simulink model "model"  (R2019b)
settings: Solver=VariableStepAuto  StartTime=0.0  StopTime=20.0  RelTol=1e-3
settings Model: Creator=szymo  LastModifiedBy=szymo

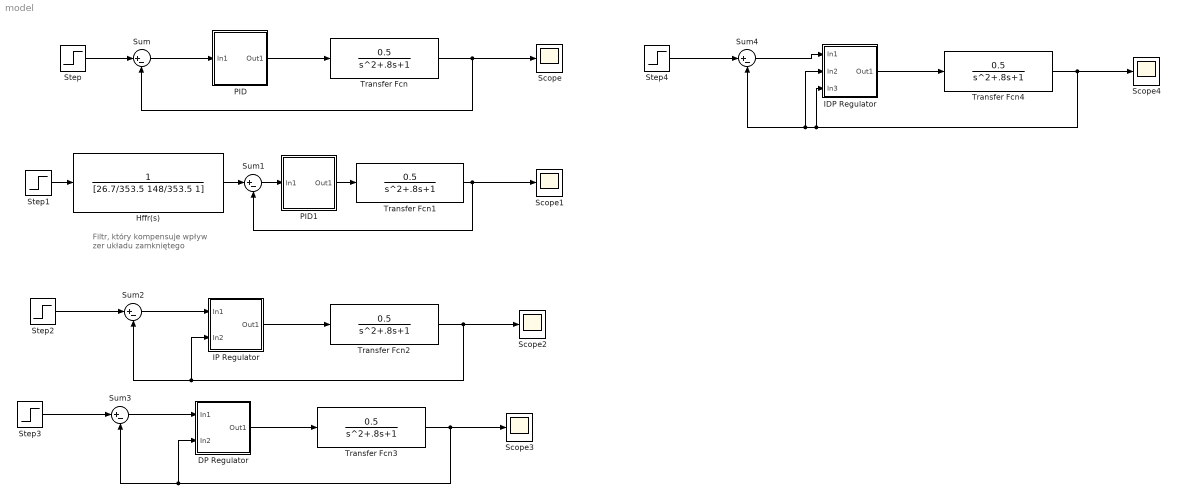
== system model ==
  note: Filtr, który kompensuje wpływ
      | zer układu zamkniętego
  DP Regulator : Subsystem
  Hffr(s) : TransferFcn  Denominator=[26.7/353.5 148/353.5 1]
  IDP Regulator : Subsystem
  IP Regulator : Subsystem
  PID : Subsystem
  PID1 : Subsystem
  Scope{,1..4} (5 alike) : Scope
  Step{,1..4} (5 alike) : Step  SampleTime=0
  Sum{,1..4} (5 alike) : Sum  Inputs=|+-
  Transfer Fcn{,1..4} (5 alike) : TransferFcn  Numerator=[0.5]  Denominator=[1 .8 1]
  wires:
  Transfer Fcn/1 -> Sum/2, Scope/1
  PID/1(Out1) -> Transfer Fcn/1
  Sum/1 -> PID/1(In1)
  Step/1 -> Sum/1
  Transfer Fcn1/1 -> Sum1/2, Scope1/1
  Sum1/1 -> PID1/1(In1)
  PID1/1(Out1) -> Transfer Fcn1/1
  Step1/1 -> Hffr(s)/1
  Hffr(s)/1 -> Sum1/1
  Step2/1 -> Sum2/1
  Sum2/1 -> IP Regulator/1(In1)
  IP Regulator/1(Out1) -> Transfer Fcn2/1
  Transfer Fcn2/1 -> IP Regulator/2(In2), Sum2/2, Scope2/1
  Step3/1 -> Sum3/1
  Transfer Fcn3/1 -> DP Regulator/2(In2), Sum3/2, Scope3/1
  Sum3/1 -> DP Regulator/1(In1)
  DP Regulator/1(Out1) -> Transfer Fcn3/1
  Sum4/1 -> IDP Regulator/1(In1)
  IDP Regulator/1(Out1) -> Transfer Fcn4/1
  Step4/1 -> Sum4/1
  Transfer Fcn4/1 -> IDP Regulator/3(In3), IDP Regulator/2(In2), Sum4/2, Scope4/1

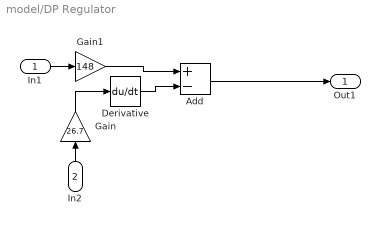
== system model/DP Regulator ==
  In1 : Inport
  In2 : Inport  Port=2
  Add : Sum  Inputs=+-
  Derivative : Derivative
  Gain : Gain  Gain=26.7
  Gain1 : Gain  Gain=148
  Out1 : Outport
  wires:
  In2/1 -> Gain/1
  Gain1/1 -> Add/1
  In1/1 -> Gain1/1
  Add/1 -> Out1/1
  Derivative/1 -> Add/2
  Gain/1 -> Derivative/1

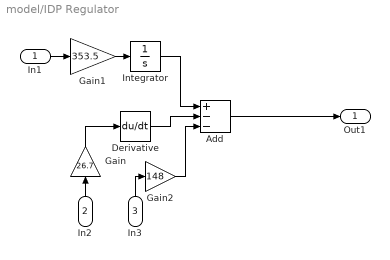
== system model/IDP Regulator ==
  In1 : Inport
  In2 : Inport  Port=2
  In3 : Inport  Port=3
  Add : Sum  Inputs=+--
  Derivative : Derivative
  Gain : Gain  Gain=26.7
  Gain1 : Gain  Gain=353.5
  Gain2 : Gain  Gain=148
  Integrator : Integrator
  Out1 : Outport
  wires:
  In2/1 -> Gain/1
  Add/1 -> Out1/1
  Derivative/1 -> Add/2
  Gain/1 -> Derivative/1
  In3/1 -> Gain2/1
  Gain2/1 -> Add/3
  In1/1 -> Gain1/1
  Gain1/1 -> Integrator/1
  Integrator/1 -> Add/1

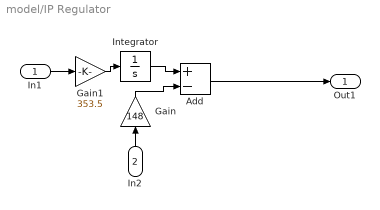
== system model/IP Regulator ==
  In1 : Inport
  In2 : Inport  Port=2
  Add : Sum  Inputs=+-
  Gain : Gain  Gain=148
  Gain1 : Gain  Gain=353.5
  Integrator : Integrator
  Out1 : Outport
  wires:
  In2/1 -> Gain/1
  Gain/1 -> Add/2
  Gain1/1 -> Integrator/1
  Integrator/1 -> Add/1
  In1/1 -> Gain1/1
  Add/1 -> Out1/1

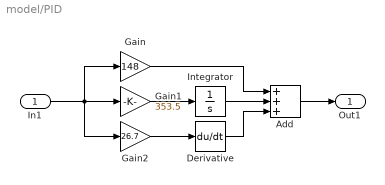
== system model/PID ==
  In1 : Inport
  Add : Sum  Inputs=+++
  Derivative : Derivative
  Gain : Gain  Gain=148
  Gain1 : Gain  Gain=353.5
  Gain2 : Gain  Gain=26.7
  Integrator : Integrator
  Out1 : Outport
  wires:
  Add/1 -> Out1/1
  Gain/1 -> Add/1
  Gain2/1 -> Derivative/1
  In1/1 -> Gain2/1, Gain/1, Gain1/1
  Derivative/1 -> Add/3
  Gain1/1 -> Integrator/1
  Integrator/1 -> Add/2

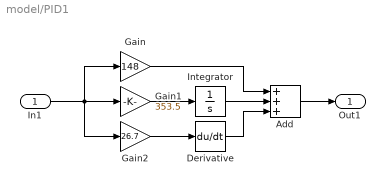
== system model/PID1 ==
  In1 : Inport
  Add : Sum  Inputs=+++
  Derivative : Derivative
  Gain : Gain  Gain=148
  Gain1 : Gain  Gain=353.5
  Gain2 : Gain  Gain=26.7
  Integrator : Integrator
  Out1 : Outport
  wires:
  Add/1 -> Out1/1
  Gain/1 -> Add/1
  Gain2/1 -> Derivative/1
  In1/1 -> Gain2/1, Gain/1, Gain1/1
  Derivative/1 -> Add/3
  Gain1/1 -> Integrator/1
  Integrator/1 -> Add/2
